simulink model "sampleModel1659_1_sub"  (R2023a)
settings: Solver=VariableStepAuto  StartTime=0.0  StopTime=10.0  RelTol=1e-3
libraries: hdlsllib x7, simulink x1
settings Model: Creator=user1  LastModifiedBy=user1
settings OptimizationCC: BlockReduction=off  ConditionallyExecuteInputs=off

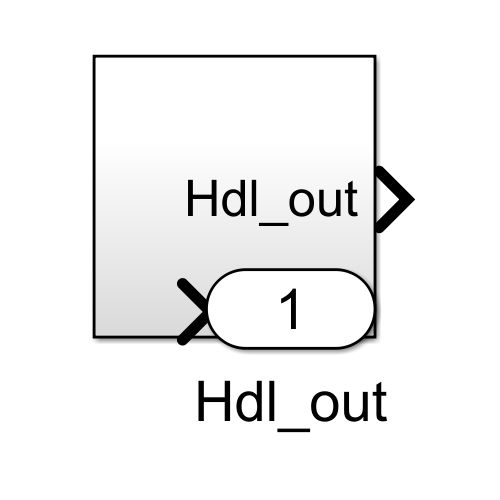
[thumbnail: Simulink's stored preview of the top-level diagram]
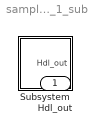
== system sampleModel1659_1_sub ==
  Subsystem : Subsystem
  Hdl_out : Outport  OutDataTypeStr=uint8

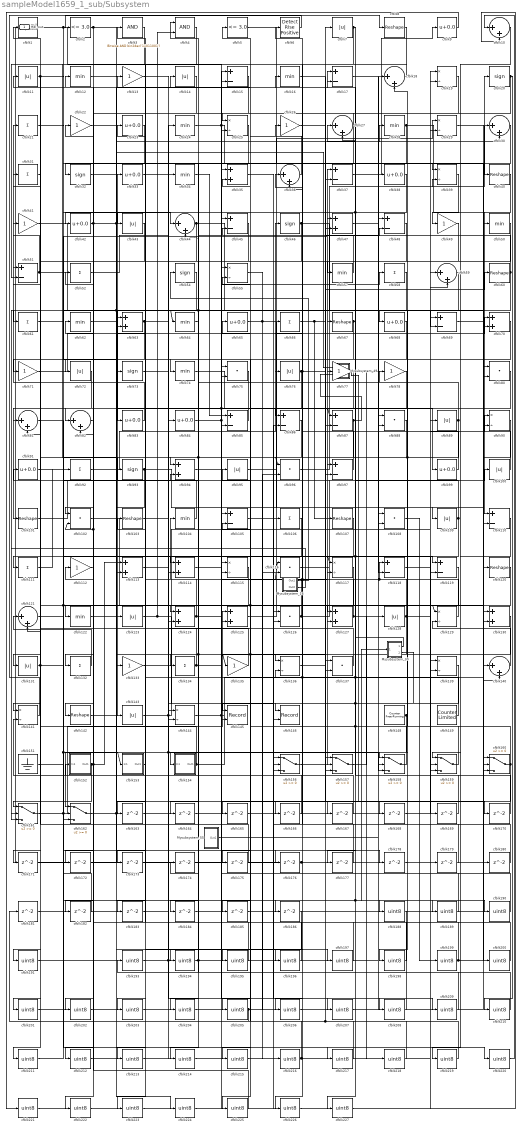
== system sampleModel1659_1_sub/Subsystem ==
  Mysubsystem_16 : Subsystem  TreatAsAtomicUnit=on  RTWFcnName=Mysubsystem_16
      settings: RTWFcnNameOpts=User specified  RTWFileNameOpts=Use function name
  Mysubsystem_30 : Subsystem  TreatAsAtomicUnit=on  RTWFcnName=Mysubsystem_30
      settings: RTWFcnNameOpts=User specified  RTWFileNameOpts=Use function name
  Mysubsystem_49 : Subsystem  TreatAsAtomicUnit=on  RTWFcnName=Mysubsystem_49
      settings: RTWFcnNameOpts=User specified  RTWFileNameOpts=Use function name
  Mysubsystem_55 : Subsystem  TreatAsAtomicUnit=on  RTWFcnName=Mysubsystem_55
      settings: RTWFcnNameOpts=User specified  RTWFileNameOpts=Use function name
  cfblk1 : hdlsllib/Logic and Bit Operations/Detect Fall Nonpositive  vinit=0  OutDataTypeStr=uint8
  cfblk{10,18,27,30,36,44,59,81..82,121,140} (11 alike) : Sum  Inputs=|++  OutDataTypeStr=uint8
  cfblk{7,11,14,43,72,76,89,95,100,109,123,128,131,143} (14 alike) : Abs  OutDataTypeStr=uint8  SaturateOnIntegerOverflow=off
  cfblk{8,40,60,67,101,103,107,120,142} (9 alike) : Reshape
  cfblk{75,80,88,96,102,108,116,126,137} (9 alike) : DotProduct  OutDataTypeStr=uint8
  cfblk{12,16,24,28,34,50,57,62,64,74,104,122} (12 alike) : MinMax  OutDataTypeStr=uint8
  cfblk{15,17,37,45,48,51,69,85..87,97,105,110,118..119} (15 alike) : Sum  Inputs=+-  OutDataTypeStr=uint8
  cfblk{21,31,52,58,61,66,92,106,111,132,134} (11 alike) : Sum  Inputs=+  OutDataTypeStr=uint8
  cfblk{13,22,26,41,49,71,77..78,112,133,135} (11 alike) : Gain  OutDataTypeStr=uint8
  cfblk{35,47,63,70,94,113..114,124..125,127,130} (11 alike) : Sum  OutDataTypeStr=uint8
  cfblk{19,25,29,39,55,90,115,117,129,136,139,141,144} (13 alike) : Product  Inputs=*/  OutDataTypeStr=uint8  RndMeth=Zero  SaturateOnIntegerOverflow=on
  cfblk145 : Record  FileSettingsInternal="{\"entries\":[{\"content\":{\"excelSettings\":{\"content\":{},\"type\":\"Streamout.ExcelSettings\"}},\"type\":\"Streamout.FileSettingStorage\",\"uuid\":\"\"}],\"packageUris\":[\"http:\\/\\/schema.mathworks.com\\/mf0\\/streamout_blocks\\/R2020a\"],\"version\":\"1.0\"}"  Layout=[1 1]  SignalsInternal="{\"entries\":[{\"content\":{\"signals\":[{\"content\":{\"blockPath\":[],\"dimensions\":[1],\"domain\":\"\",\"lineColor\":\"#a2142f\",\"plots\":[1],\"port\":1,\"signalID\":31944,\"signalName\":\"cfblk70\"},\"type\":\"RecordBlkView.Signal\",\"uuid\":\"\"},{\"content\":{\"blockPath\":[],\"dimensions\":[1],\"domain\":\"\",\"lineColor\":\"#139fff\",\"plots\":[1],\"port\":2,\"signalID\":31947,\"signalName\":\"cfblk63\"},\"type\":\"RecordBlkView.Signal\",\"uuid\":\"\"}]},\"type\":\"RecordBlkView.InputSignals\",\"uuid\":\"\"}],\"packageUris\":[\"http:\\/\\/schema.mathworks.com\\/mf0\\/streamout_blocks\\/R2020a\"],\"version\":\"1.0\"}"  VisualizationBindings="{\"xyplotplugin\":{\"info\":[{\"series\":[{\"bindingParametersList\":[{\"parameter\":\"X-Axis\",\"signalID\":31944,\"signalName\":\"cfblk70\"},{\"parameter\":\"Y-Axis\",\"signalID\":31947,\"signalName\":\"cfblk63\"}],\"seriesID\":21604}],\"subplotID\":1}]}}"  CompatibilityTag=XY  st=-1
  cfblk146 : Record  FileSettingsInternal="{\"entries\":[{\"content\":{\"excelSettings\":{\"content\":{},\"type\":\"Streamout.ExcelSettings\"}},\"type\":\"Streamout.FileSettingStorage\",\"uuid\":\"\"}],\"packageUris\":[\"http:\\/\\/schema.mathworks.com\\/mf0\\/streamout_blocks\\/R2020a\"],\"version\":\"1.0\"}"  Layout=[1 1]  SignalsInternal="{\"entries\":[{\"content\":{\"signals\":[{\"content\":{\"blockPath\":[],\"dimensions\":[1],\"domain\":\"\",\"lineColor\":\"#a2142f\",\"plots\":[1],\"port\":1,\"signalID\":31936,\"signalName\":\"cfblk78\"},\"type\":\"RecordBlkView.Signal\",\"uuid\":\"\"},{\"content\":{\"blockPath\":[],\"dimensions\":[1],\"domain\":\"\",\"lineColor\":\"#139fff\",\"plots\":[1],\"port\":2,\"signalID\":31939,\"signalName\":\"cfblk24\"},\"type\":\"RecordBlkView.Signal\",\"uuid\":\"\"}]},\"type\":\"RecordBlkView.InputSignals\",\"uuid\":\"\"}],\"packageUris\":[\"http:\\/\\/schema.mathworks.com\\/mf0\\/streamout_blocks\\/R2020a\"],\"version\":\"1.0\"}"  VisualizationBindings="{\"xyplotplugin\":{\"info\":[{\"series\":[{\"bindingParametersList\":[{\"parameter\":\"X-Axis\",\"signalID\":31936,\"signalName\":\"cfblk78\"},{\"parameter\":\"Y-Axis\",\"signalID\":31939,\"signalName\":\"cfblk24\"}],\"seriesID\":15880}],\"subplotID\":1}]}}"  CompatibilityTag=XY  st=-1
  cfblk148 : hdlsllib/Sources/Counter Free-Running  NumBits=16  tsamp=-1
  cfblk149 : hdlsllib/Sources/Counter Limited  uplimit=7  tsamp=-1
  cfblk151 : Ground
  cfblk152 : Subsystem
      settings: LibrarySourceBlock=|
      | hdlsllib/Ports &
      | Subsystems/Subsystem
  cfblk153 : Subsystem
      settings: LibrarySourceBlock=|
      | hdlsllib/Ports &
      | Subsystems/Subsystem
  cfblk154 : Subsystem
      settings: LibrarySourceBlock=|
      | hdlsllib/Ports &
      | Subsystems/Subsystem
  cfblk{156..162} (7 alike) : Switch  OutDataTypeStr=uint8  SaturateOnIntegerOverflow=off  InputSameDT=off
  cfblk{163..186} (24 alike) : Delay  SampleTime=1
  cfblk{188..191,193..227} (39 alike) : DataTypeConversion  OutDataTypeStr=uint8  SaturateOnIntegerOverflow=off  RndMeth=Floor
  cfblk2 : hdlsllib/Logic and Bit Operations/Compare To Constant  relop=<=  const=3.0  OutDataTypeStr=uint8
  cfblk{20,32,46,54,73,93} (6 alike) : Signum
  cfblk{9,23,33,38,42,65,68,83..84,91,99} (11 alike) : Bias  Bias=0.0  SaturateOnIntegerOverflow=off
  cfblk3 : simulink/Logic and Bit Operations/Bitwise Operator  logicop=AND  UseBitMask=on  BitMask=bin2dec('11011001')  BitMaskRealWorld=Stored Integer
      settings: LibrarySourceBlock=|
      | hdlsllib/Logic and Bit
      | Operations/Bitwise
      | Operator
  cfblk4 : Logic  AllPortsSameDT=off  OutDataTypeStr=boolean
  cfblk5 : hdlsllib/Logic and Bit Operations/Compare To Constant  relop=<=  const=3.0  OutDataTypeStr=uint8
  cfblk6 : hdlsllib/Logic and Bit Operations/Detect Rise Positive  vinit=0  OutDataTypeStr=uint8
  Hdl_out : Outport  OutDataTypeStr=uint8
  wires:
  cfblk124/1 -> cfblk117/2, cfblk104/1
  cfblk157/1 -> cfblk128/1
  cfblk25/1 -> cfblk32/1
  cfblk34/1 -> cfblk85/1
  cfblk95/1 -> cfblk109/1
  cfblk36/1 -> cfblk14/1
  cfblk20/1 -> cfblk210/1, cfblk94/1
  cfblk111/1 -> cfblk92/1
  cfblk18/1 -> cfblk143/1
  cfblk40/1 -> cfblk110/1
  cfblk161/1 -> cfblk100/1, cfblk125/1
  cfblk60/1 -> cfblk198/1, cfblk26/1
  cfblk99/1 -> cfblk37/1
  cfblk141/1 -> cfblk8/1
  cfblk37/1 -> cfblk9/1
  cfblk108/1 -> cfblk199/1
  cfblk125/1 -> cfblk29/1
  cfblk72/1 -> cfblk101/1
  cfblk55/1 -> cfblk216/1
  cfblk11/1 -> cfblk44/1, cfblk161/1
  cfblk101/1 -> cfblk33/1
  cfblk96/1 -> cfblk20/1
  cfblk156/1 -> cfblk67/1
  cfblk76/1 -> cfblk173/1, cfblk226/1, cfblk170/1
  cfblk15/1 -> cfblk82/1
  cfblk93/1 -> cfblk120/1, cfblk123/1
  cfblk32/1 -> cfblk85/2, cfblk64/1
  cfblk41/1 -> cfblk83/1
  cfblk148/1 -> cfblk78/1, cfblk162/1
  cfblk10/1 -> cfblk219/1
  cfblk88/1 -> cfblk191/1
  cfblk117/1 -> cfblk131/1, cfblk185/1, cfblk135/1
  cfblk83/1 -> cfblk21/1
  cfblk43/1 -> cfblk111/1
  cfblk2/1 -> cfblk189/1, cfblk122/1
  cfblk137/1 -> cfblk97/1
  cfblk57/1 -> cfblk11/1
  cfblk65/1 -> cfblk116/2, cfblk140/1
  cfblk85/1 -> cfblk81/1
  cfblk7/1 -> cfblk57/1, cfblk43/1
  cfblk104/1 -> cfblk51/1
  cfblk74/1 -> cfblk99/1
  cfblk149/1 -> cfblk77/1, cfblk103/1, cfblk36/1
  cfblk112/1 -> cfblk22/1
  cfblk154/1(Out1) -> cfblk31/1, cfblk59/1
  cfblk92/1 -> cfblk46/1
  cfblk29/1 -> cfblk40/1
  cfblk81/1 -> cfblk176/1, cfblk153/1(In1)
  cfblk39/1 -> cfblk49/1
  cfblk16/1 -> cfblk157/1
  cfblk5/1 -> cfblk50/1
  cfblk102/1 -> cfblk140/2
  cfblk1/1 -> cfblk37/2, cfblk125/2
  cfblk54/1 -> cfblk161/2
  cfblk136/1 -> cfblk48/2
  cfblk3/1 -> cfblk42/1
  cfblk132/1 -> cfblk121/1
  cfblk131/1 -> cfblk201/1, cfblk186/1
  cfblk159/1 -> cfblk95/1
  cfblk52/1 -> cfblk24/1
  cfblk42/1 -> cfblk102/1, cfblk124/2, cfblk16/1
  cfblk28/1 -> cfblk87/2, cfblk130/1
  cfblk153/1(Out1) -> cfblk23/1
  cfblk63/1 -> cfblk145/2, cfblk81/2
  cfblk77/1 -> cfblk195/1, cfblk218/1, cfblk18/1
  cfblk129/1 -> cfblk118/1, cfblk13/1, cfblk76/1
  cfblk91/1 -> cfblk118/2
  cfblk160/1 -> cfblk206/1, cfblk18/2
  cfblk97/1 -> cfblk36/2
  cfblk30/1 -> cfblk142/1
  cfblk6/1 -> cfblk2/1
  cfblk27/1 -> cfblk124/1, cfblk25/1
  cfblk24/1 -> cfblk146/2, cfblk39/1
  cfblk127/1 -> cfblk6/1, cfblk39/2
  cfblk51/1 -> cfblk113/2, cfblk41/1
  cfblk134/1 -> cfblk207/1, cfblk91/1
  cfblk45/1 -> cfblk194/1
  cfblk94/1 -> cfblk137/2
  cfblk143/1 -> cfblk127/2, cfblk69/1
  cfblk80/1 -> cfblk205/1
  cfblk84/1 -> cfblk158/3, cfblk17/2, cfblk87/1
  cfblk26/1 -> cfblk97/2
  cfblk31/1 -> cfblk61/1
  cfblk44/1 -> cfblk82/2, cfblk69/2
  cfblk100/1 -> cfblk90/1
  cfblk4/1 -> cfblk51/2
  cfblk109/1 -> cfblk215/1, cfblk27/2
  cfblk61/1 -> cfblk68/1
  cfblk144/1 -> cfblk30/2, cfblk30/1
  cfblk158/1 -> cfblk17/1, cfblk116/1, cfblk66/1
  cfblk23/1 -> cfblk132/1
  cfblk122/1 -> cfblk70/1
  cfblk21/1 -> cfblk73/1
  cfblk121/1 -> cfblk47/1, cfblk129/1
  cfblk71/1 -> cfblk15/2
  cfblk8/1 -> cfblk86/1
  cfblk87/1 -> cfblk136/1, Mysubsystem_49/2(In2)
  cfblk103/1 -> cfblk190/1, cfblk157/3
  cfblk66/1 -> cfblk107/1, cfblk60/1
  cfblk59/1 -> cfblk164/1, cfblk144/2
  cfblk116/1 -> cfblk38/1
  cfblk128/1 -> cfblk90/2, cfblk63/1, cfblk184/1, cfblk183/1
  cfblk78/1 -> cfblk146/1
  cfblk17/1 -> cfblk119/1
  cfblk142/1 -> cfblk28/1
  cfblk47/1 -> cfblk119/2
  cfblk140/1 -> cfblk129/2
  cfblk90/1 -> cfblk160/2
  cfblk114/1 -> cfblk58/1
  cfblk68/1 -> cfblk74/1
  cfblk70/1 -> cfblk145/1
  cfblk46/1 -> cfblk203/1, cfblk70/2
  cfblk152/1(Out1) -> cfblk171/1, cfblk52/1, cfblk113/1
  cfblk89/1 -> cfblk4/1, cfblk96/1, cfblk158/1
  cfblk126/1 -> cfblk94/2, cfblk89/1
  cfblk133/1 -> cfblk156/1
  cfblk110/1 -> cfblk159/1
  cfblk50/1 -> cfblk121/2
  cfblk38/1 -> cfblk177/1, cfblk72/1
  cfblk86/1 -> cfblk163/1, cfblk154/1(In1)
  cfblk48/1 -> cfblk93/1
  cfblk58/1 -> cfblk141/1
  cfblk135/1 -> cfblk112/1
  cfblk120/1 -> cfblk133/1
  cfblk123/1 -> cfblk4/2, cfblk156/3
  cfblk64/1 -> cfblk114/1
  cfblk162/1 -> cfblk224/1, cfblk166/1
  cfblk107/1 -> cfblk134/1
  cfblk67/1 -> cfblk127/1, cfblk71/1
  cfblk163/1 -> cfblk29/2
  cfblk164/1 -> cfblk25/2
  cfblk165/1 -> cfblk86/2
  cfblk166/1 -> cfblk141/2
  cfblk73/1 -> cfblk167/1
  cfblk167/1 -> cfblk15/1
  cfblk113/1 -> cfblk168/1
  cfblk168/1 -> cfblk59/2
  cfblk118/1 -> cfblk169/1
  cfblk169/1 -> cfblk27/1
  cfblk170/1 -> cfblk48/1
  cfblk171/1 -> cfblk63/2
  cfblk49/1 -> cfblk172/1
  cfblk172/1 -> cfblk157/2
  cfblk173/1 -> cfblk158/2
  cfblk174/1 -> cfblk126/2
  cfblk119/1 -> cfblk175/1
  cfblk175/1 -> cfblk1/1
  cfblk176/1 -> Hdl_out/1, cfblk159/3
  cfblk177/1 -> cfblk156/2
  cfblk33/1 -> cfblk178/1
  cfblk178/1 -> cfblk160/3
  cfblk179/1 -> cfblk136/2
  cfblk180/1 -> cfblk159/2
  cfblk181/1 -> cfblk144/1
  cfblk14/1 -> cfblk182/1
  cfblk182/1 -> cfblk162/2
  cfblk183/1 -> cfblk114/2
  cfblk184/1 -> cfblk130/2
  cfblk185/1 -> cfblk110/2
  cfblk35/1 -> cfblk188/1
  cfblk189/1 -> cfblk35/1
  cfblk190/1 -> cfblk35/2
  cfblk191/1 -> cfblk34/1, cfblk47/2
  cfblk188/1 -> cfblk193/1
  cfblk193/1 -> cfblk88/2
  cfblk194/1 -> cfblk7/1, cfblk44/2
  cfblk195/1 -> cfblk45/1
  cfblk196/1 -> cfblk45/2
  cfblk62/1 -> cfblk197/1
  cfblk197/1 -> cfblk3/1
  cfblk198/1 -> cfblk62/1
  cfblk199/1 -> cfblk180/1, cfblk12/1, cfblk102/2
  cfblk69/1 -> cfblk200/1
  cfblk200/1 -> cfblk108/1
  cfblk201/1 -> cfblk108/2
  cfblk75/1 -> cfblk202/1
  cfblk202/1 -> cfblk160/1
  cfblk203/1 -> cfblk75/1
  cfblk204/1 -> cfblk75/2
  cfblk205/1 -> cfblk96/2, cfblk181/1
  cfblk206/1 -> cfblk80/1
  cfblk207/1 -> cfblk80/2
  cfblk105/1 -> cfblk208/1
  cfblk208/1 -> cfblk174/1
  cfblk13/1 -> cfblk209/1
  cfblk209/1 -> cfblk105/1
  cfblk210/1 -> cfblk105/2
  cfblk106/1 -> cfblk211/1
  cfblk211/1 -> cfblk162/3
  cfblk82/1 -> cfblk212/1
  cfblk212/1 -> cfblk106/1
  cfblk19/1 -> cfblk213/1
  cfblk213/1 -> cfblk84/1
  cfblk130/1 -> cfblk214/1
  cfblk214/1 -> cfblk19/1
  cfblk215/1 -> cfblk19/2
  cfblk216/1 -> cfblk65/1, cfblk179/1
  cfblk12/1 -> cfblk217/1
  cfblk217/1 -> cfblk55/1
  cfblk218/1 -> cfblk55/2
  cfblk219/1 -> cfblk137/1, cfblk5/1
  cfblk151/1 -> cfblk220/1
  cfblk220/1 -> cfblk10/1
  cfblk9/1 -> cfblk221/1
  cfblk221/1 -> cfblk10/2
  cfblk115/1 -> cfblk222/1
  cfblk222/1 -> cfblk126/1
  cfblk186/1 -> cfblk223/1
  cfblk223/1 -> cfblk115/1
  cfblk224/1 -> cfblk115/2
  cfblk139/1 -> cfblk225/1
  cfblk225/1 -> cfblk152/1(In1)
  cfblk226/1 -> cfblk139/1
  cfblk227/1 -> cfblk139/2
  Mysubsystem_16/1(Out1) -> cfblk54/1
  Mysubsystem_16/2(Out2) -> cfblk161/3
  Mysubsystem_30/2(Out2) -> cfblk196/1, cfblk227/1, Mysubsystem_30/1(In1)
  Mysubsystem_30/1(Out1) -> cfblk117/1, cfblk204/1
  cfblk22/1 -> Mysubsystem_49/1(In1)
  Mysubsystem_49/1(Out1) -> cfblk165/1
  Mysubsystem_55/1(Out1) -> cfblk88/1

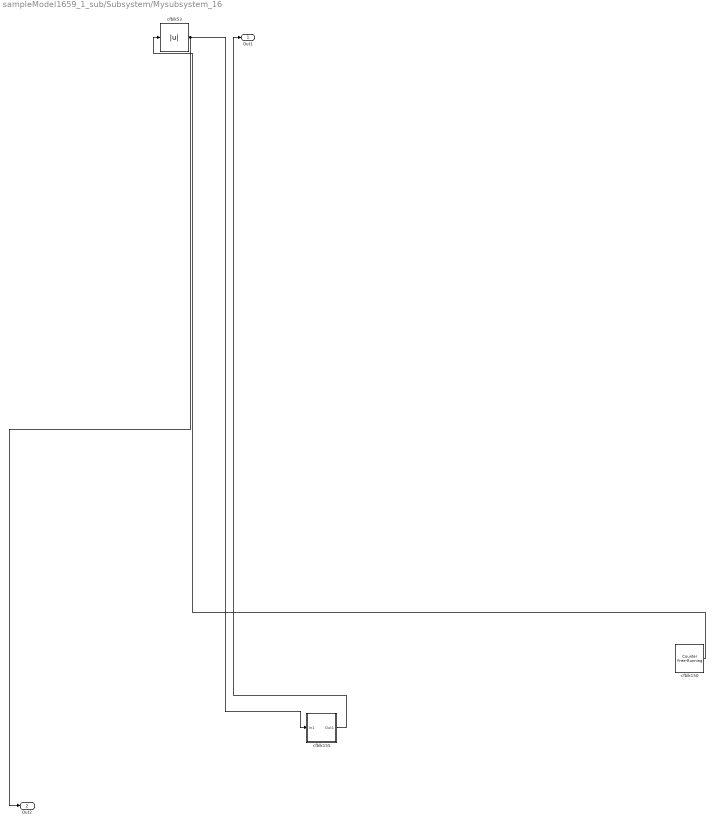
== system sampleModel1659_1_sub/Subsystem/Mysubsystem_16 ==
  cfblk150 : hdlsllib/Sources/Counter Free-Running  NumBits=16  tsamp=-1
  cfblk155 : Subsystem
      settings: LibrarySourceBlock=|
      | hdlsllib/Ports &
      | Subsystems/Subsystem
  cfblk53 : Abs  SaturateOnIntegerOverflow=off
  Out1 : Outport
  Out2 : Outport  Port=2
  wires:
  cfblk155/1(Out1) -> Out1/1
  cfblk53/1 -> cfblk155/1(In1), Out2/1
  cfblk150/1 -> cfblk53/1

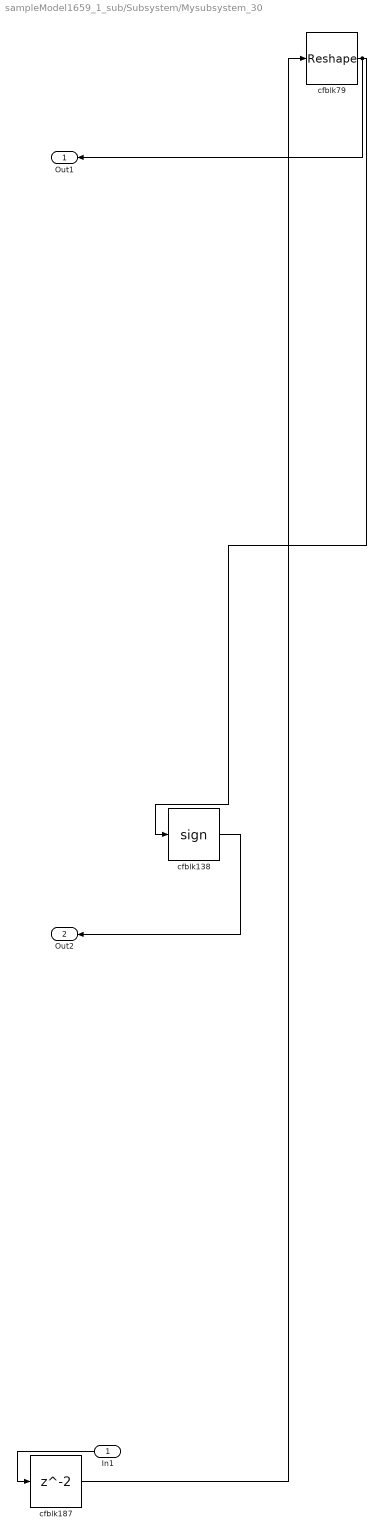
== system sampleModel1659_1_sub/Subsystem/Mysubsystem_30 ==
  In1 : Inport
  cfblk138 : Signum
  cfblk187 : Delay  SampleTime=1
  cfblk79 : Reshape
  Out1 : Outport
  Out2 : Outport  Port=2
  wires:
  In1/1 -> cfblk187/1
  cfblk138/1 -> Out2/1
  cfblk187/1 -> cfblk79/1
  cfblk79/1 -> cfblk138/1, Out1/1

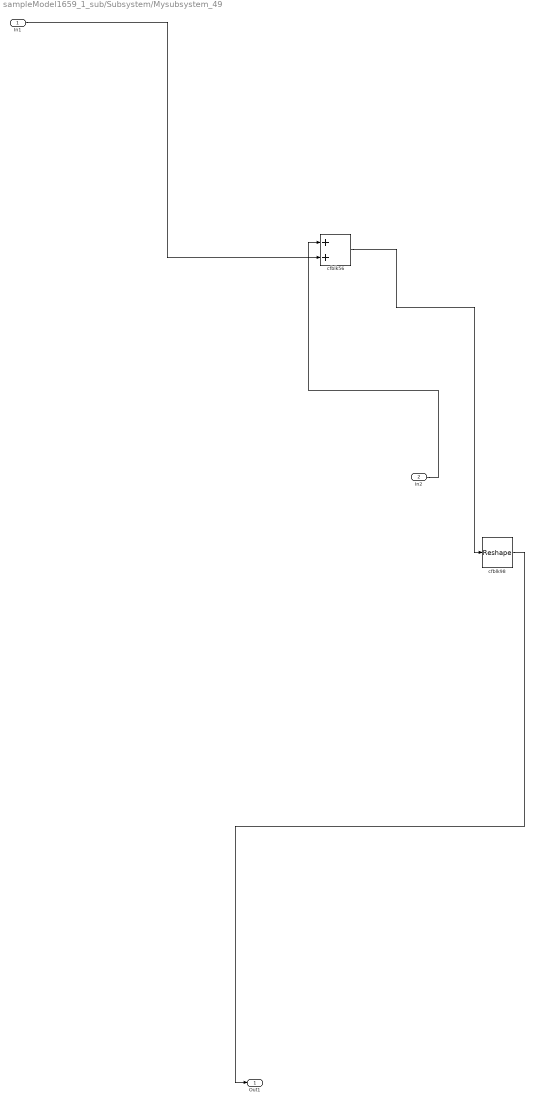
== system sampleModel1659_1_sub/Subsystem/Mysubsystem_49 ==
  In1 : Inport
  In2 : Inport  Port=2
  cfblk56 : Sum
  cfblk98 : Reshape
  Out1 : Outport
  wires:
  In1/1 -> cfblk56/2
  cfblk98/1 -> Out1/1
  In2/1 -> cfblk56/1
  cfblk56/1 -> cfblk98/1

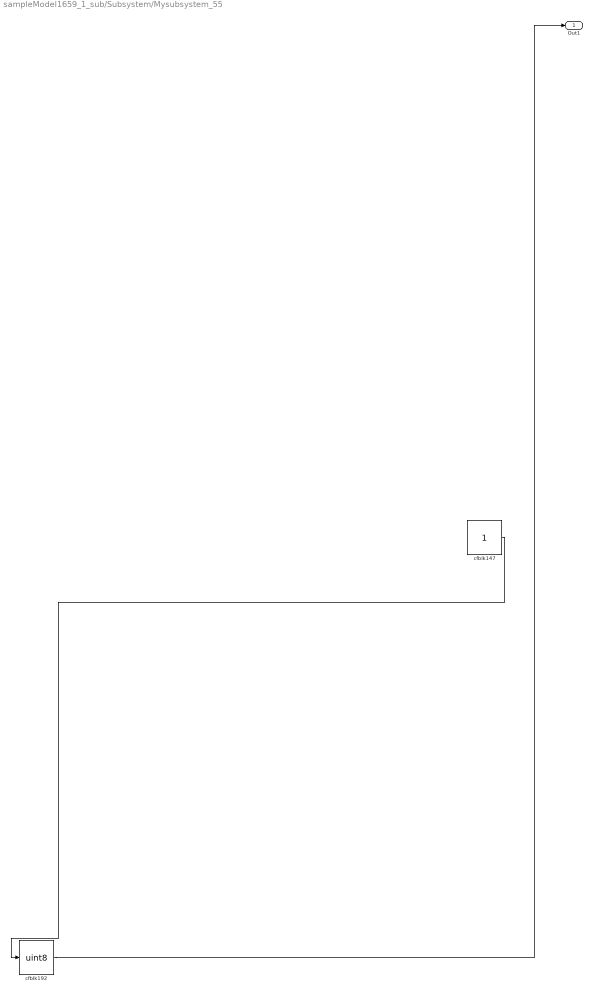
== system sampleModel1659_1_sub/Subsystem/Mysubsystem_55 ==
  cfblk147 : Constant  SampleTime=-1
  cfblk192 : DataTypeConversion  OutDataTypeStr=uint8  SaturateOnIntegerOverflow=off  RndMeth=Floor
  Out1 : Outport
  wires:
  cfblk192/1 -> Out1/1
  cfblk147/1 -> cfblk192/1

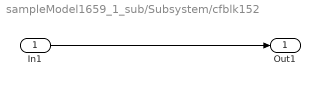
== system sampleModel1659_1_sub/Subsystem/cfblk152 ==
  In1 : Inport
  Out1 : Outport
  wires:
  In1/1 -> Out1/1

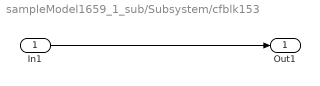
== system sampleModel1659_1_sub/Subsystem/cfblk153 ==
  In1 : Inport
  Out1 : Outport
  wires:
  In1/1 -> Out1/1

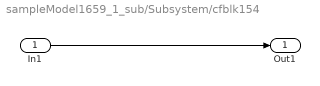
== system sampleModel1659_1_sub/Subsystem/cfblk154 ==
  In1 : Inport
  Out1 : Outport
  wires:
  In1/1 -> Out1/1

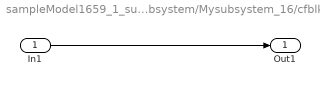
== system sampleModel1659_1_sub/Subsystem/Mysubsystem_16/cfblk155 ==
  In1 : Inport
  Out1 : Outport
  wires:
  In1/1 -> Out1/1
